simulink model "model8Krata"  (Simulink 6.6)
settings: Solver=ode45  StartTime=0.0  StopTime=250  MaxStep=0.01  MinStep=0.001  RelTol=1e-6
values from neighbouring files (symbols this model uses):
  a1 = w1/w0    (= 84)    [dane8Krata.m]
  a2 = w2/w0    (= 273)    [dane8Krata.m]
  a3 = 1/w0    (= 180)    [dane8Krata.m]
  b0 = d12*d23 / (C1*w0)    (= 3)    [dane8Krata.m]
  p0 = 1    [dane8Krata.m]
undefined symbols (not defined in the file or in its folder): kp, Td, Ti
libraries: simulink_extras x1
settings Model: Creator=Administrator  LastModifiedBy=Damian
settings DataIOCC: LimitDataPoints=off
settings DebuggingCC: SignalResolutionControl=TryResolveAllWithWarning  MultiTaskDSMMsg=warning  MultiTaskCondExecSysMsg=none  StrictBusMsg=None
settings RTWCC: IncludeERTFirstTime=on

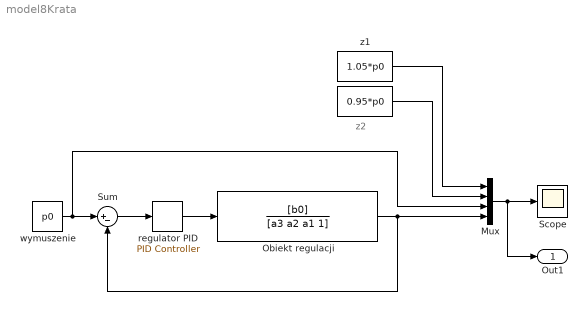
== system model8Krata ==
  note: z2
  " " : Constant  Value=0.95*p0
  Mux : Mux
  Obiekt regulacji : TransferFcn  Numerator=[b0]  Denominator=[a3 a2 a1 1]
  Scope : Scope
      settings: YMin=-100000  YMax=100000
  Sum : Sum  Inputs=|+-
  regulator PID : simulink_extras/Additional Linear/PID Controller  SystemSampleTime=-1  P=kp  I=kp/Ti  D=Td*kp
  wymuszenie : Constant  Value=p0
  z1 : Constant  Value=1.05*p0
  Out1 : Outport
  wires:
  wymuszenie/1 -> Sum/1, Mux/3
  Mux/1 -> Scope/1, Out1/1
  Sum/1 -> regulator PID/1
  regulator PID/1 -> Obiekt regulacji/1
  Obiekt regulacji/1 -> Sum/2, Mux/4
  " "/1 -> Mux/2
  z1/1 -> Mux/1
